simulink subsystem "AeroPropRefFranc"  (R2024b)
settings: Solver=VariableStepAuto  StartTime=0.0  StopTime=10.0  RelTol=1e-3
undefined symbols (not defined in the file or in its folder): ess, Force_b, Fprop_r, geom, H_b, Hdot_b, Moment_b, mot, mot2, mot3, mot4, Mprop_r, propel, propel2, propel3, propel4, pxf_diagram_options, SimIn, SimPar, tc, tc2, tc3, tc4
libraries: simulink x8, slpidlib x4, starslibAxisTransformations x2, libAxisTransformations x2
(part 4 of 10)

== system AeroPropRefFranc/Propulsion and Aerodynamic Forces and Moments/S-Function/Battery Model/powerplant/ess (battery)1/plant/parameter_out ==
  inport-ess_plant_soc_simu : Inport
  inport-ess_plant_curr_out_simu : Inport  Port=2
  inport-ess_plant_volt_out_simu : Inport  Port=3
  inport-ess_plant_voc_simu : Inport  Port=4
  inport-ess_plant_rint_simu : Inport  Port=5
  inport-ess_plant_rpol1_simu : Inport  Port=6
  inport-ess_plant_rpol2_simu : Inport  Port=7
  inport-ess_plant_curr_pol1_simu : Inport  Port=8
  inport-ess_plant_curr_pol2_simu : Inport  Port=9
  inport-ess_plant_heat_out_simu : Inport  Port=10
  inport-ess_plant_impedance_simu : Inport  Port=11
  Ground_1 : Ground
  Toworkspace-ess_plant_curr_out_simu : ToWorkspace  VariableName=ess_plant_curr_out_simu  SampleTime=pxf_diagram_options.workspace_sample_time
      settings: Decimation=pxf_diagram_options.decimation
  Toworkspace-ess_plant_curr_pol1_simu : ToWorkspace  VariableName=ess_plant_curr_pol1_simu  SampleTime=pxf_diagram_options.workspace_sample_time
      settings: Decimation=pxf_diagram_options.decimation
  Toworkspace-ess_plant_curr_pol2_simu : ToWorkspace  VariableName=ess_plant_curr_pol2_simu  SampleTime=pxf_diagram_options.workspace_sample_time
      settings: Decimation=pxf_diagram_options.decimation
  Toworkspace-ess_plant_heat_out_simu : ToWorkspace  VariableName=ess_plant_heat_out_simu  SampleTime=pxf_diagram_options.workspace_sample_time
      settings: Decimation=pxf_diagram_options.decimation
  Toworkspace-ess_plant_impedance_simu : ToWorkspace  VariableName=ess_plant_impedance_simu  SampleTime=pxf_diagram_options.workspace_sample_time
      settings: Decimation=pxf_diagram_options.decimation
  Toworkspace-ess_plant_rint_simu : ToWorkspace  VariableName=ess_plant_rint_simu  SampleTime=pxf_diagram_options.workspace_sample_time
      settings: Decimation=pxf_diagram_options.decimation
  Toworkspace-ess_plant_rpol1_simu : ToWorkspace  VariableName=ess_plant_rpol1_simu  SampleTime=pxf_diagram_options.workspace_sample_time
      settings: Decimation=pxf_diagram_options.decimation
  Toworkspace-ess_plant_rpol2_simu : ToWorkspace  VariableName=ess_plant_rpol2_simu  SampleTime=pxf_diagram_options.workspace_sample_time
      settings: Decimation=pxf_diagram_options.decimation
  Toworkspace-ess_plant_soc_simu : ToWorkspace  VariableName=ess_plant_soc_simu  SampleTime=pxf_diagram_options.workspace_sample_time
      settings: Decimation=pxf_diagram_options.decimation
  Toworkspace-ess_plant_voc_simu : ToWorkspace  VariableName=ess_plant_voc_simu  SampleTime=pxf_diagram_options.workspace_sample_time
      settings: Decimation=pxf_diagram_options.decimation
  Toworkspace-ess_plant_volt_out_simu : ToWorkspace  VariableName=ess_plant_volt_out_simu  SampleTime=pxf_diagram_options.workspace_sample_time
      settings: Decimation=pxf_diagram_options.decimation
  create_system_info_bus : BusCreator  Inputs=3
  outport-system_info_bus : Outport
  outport-plant_bus : Outport  Port=2
  wires:
  create_system_info_bus/1 -> outport-system_info_bus/1
  inport-ess_plant_soc_simu/1 -> create_system_info_bus/1, Toworkspace-ess_plant_soc_simu/1  "ess_plant_soc_simu"
  inport-ess_plant_heat_out_simu/1 -> Toworkspace-ess_plant_heat_out_simu/1
  inport-ess_plant_impedance_simu/1 -> Toworkspace-ess_plant_impedance_simu/1
  inport-ess_plant_curr_out_simu/1 -> create_system_info_bus/2, Toworkspace-ess_plant_curr_out_simu/1  "ess_plant_curr_out_simu"
  inport-ess_plant_volt_out_simu/1 -> create_system_info_bus/3, Toworkspace-ess_plant_volt_out_simu/1  "ess_plant_volt_out_simu"
  inport-ess_plant_voc_simu/1 -> Toworkspace-ess_plant_voc_simu/1
  inport-ess_plant_rint_simu/1 -> Toworkspace-ess_plant_rint_simu/1
  inport-ess_plant_rpol1_simu/1 -> Toworkspace-ess_plant_rpol1_simu/1
  inport-ess_plant_rpol2_simu/1 -> Toworkspace-ess_plant_rpol2_simu/1
  inport-ess_plant_curr_pol1_simu/1 -> Toworkspace-ess_plant_curr_pol1_simu/1
  inport-ess_plant_curr_pol2_simu/1 -> Toworkspace-ess_plant_curr_pol2_simu/1
  Ground_1/1 -> outport-plant_bus/1

== system AeroPropRefFranc/Propulsion and Aerodynamic Forces and Moments/S-Function/Battery Model/powerplant/ess (battery)1/plant/parameter_selection ==

== system AeroPropRefFranc/Propulsion and Aerodynamic Forces and Moments/S-Function/Battery Model/powerplant/mot/ctrl/cmd ==
  inport-main_info_bus-1 : Inport
  aInport--2 : Inport  Port=2
  aInport--3 : Inport  Port=3
  aInport--4 : Inport  Port=4
  Terminator_1 : Terminator
  Terminator_2 : Terminator
  Terminator_3 : Terminator
  mot_ctrl_cmd_map_Pelec_funTW_volt_in : Subsystem
  parameter_out : Subsystem
  parameter_selection : Subsystem
  outport-system_info_bus : Outport
  wires:
  aInport--4/1 -> Terminator_3/1
  aInport--3/1 -> Terminator_2/1
  aInport--2/1 -> Terminator_1/1
  parameter_selection/4(outport-mot_ctrl_cstr_trq_max_neg_simu-4) -> mot_ctrl_cmd_map_Pelec_funTW_volt_in/4(mot_ctrl_cstr_trq_max_neg_simu)
  parameter_selection/3(outport-mot_ctrl_cstr_trq_max_pos_simu-3) -> mot_ctrl_cmd_map_Pelec_funTW_volt_in/3(mot_ctrl_cstr_trq_max_pos_simu)
  parameter_selection/2(outport-mot_ctrl_trs_trq_simu-2) -> mot_ctrl_cmd_map_Pelec_funTW_volt_in/2(mot_ctrl_trs_trq_simu)
  parameter_selection/1(outport-mot_plant_spd_out_simu-1) -> mot_ctrl_cmd_map_Pelec_funTW_volt_in/1(mot_plant_spd_out_simu)
  mot_ctrl_cmd_map_Pelec_funTW_volt_in/1(mot_ctrl_cmd_simu) -> parameter_out/1(inport-mot_ctrl_cmd_simu)
  parameter_out/1(outport-system_info_bus) -> outport-system_info_bus/1
  inport-main_info_bus-1/1 -> parameter_selection/1(inport-main_info_bus-1)

== system AeroPropRefFranc/Propulsion and Aerodynamic Forces and Moments/S-Function/Battery Model/powerplant/mot/ctrl/cstr ==
  inport-main_info_bus-1 : Inport
  aInport--2 : Inport  Port=2
  aInport--3 : Inport  Port=3
  Terminator_1 : Terminator
  Terminator_2 : Terminator
  mot_ctrl_cstr_map_Pelec_funTW_volt_in : Subsystem
  parameter_out : Subsystem
  parameter_selection : Subsystem
  outport-system_info_bus : Outport
  outport-cstr_bus : Outport  Port=2
  wires:
  aInport--3/1 -> Terminator_2/1
  aInport--2/1 -> Terminator_1/1
  parameter_selection/2(outport-mot_plant_temp_coeff_simu-2) -> mot_ctrl_cstr_map_Pelec_funTW_volt_in/2(mot_plant_temp_coeff_simu)
  parameter_selection/1(outport-mot_plant_spd_out_simu-1) -> mot_ctrl_cstr_map_Pelec_funTW_volt_in/1(mot_plant_spd_out_simu)
  mot_ctrl_cstr_map_Pelec_funTW_volt_in/7(mot_ctrl_cstr_temp_coeff_simu) -> parameter_out/7(inport-mot_ctrl_cstr_temp_coeff_simu)
  mot_ctrl_cstr_map_Pelec_funTW_volt_in/6(mot_ctrl_cstr_trq_cont_neg_simu) -> parameter_out/6(inport-mot_ctrl_cstr_trq_cont_neg_simu)
  mot_ctrl_cstr_map_Pelec_funTW_volt_in/5(mot_ctrl_cstr_trq_cont_pos_simu) -> parameter_out/5(inport-mot_ctrl_cstr_trq_cont_pos_simu)
  mot_ctrl_cstr_map_Pelec_funTW_volt_in/4(mot_ctrl_cstr_trq_max_neg_simu) -> parameter_out/4(inport-mot_ctrl_cstr_trq_max_neg_simu)
  mot_ctrl_cstr_map_Pelec_funTW_volt_in/3(mot_ctrl_cstr_trq_pk_neg_simu) -> parameter_out/3(inport-mot_ctrl_cstr_trq_pk_neg_simu)
  mot_ctrl_cstr_map_Pelec_funTW_volt_in/2(mot_ctrl_cstr_trq_max_pos_simu) -> parameter_out/2(inport-mot_ctrl_cstr_trq_max_pos_simu)
  mot_ctrl_cstr_map_Pelec_funTW_volt_in/1(mot_ctrl_cstr_trq_pk_pos_simu) -> parameter_out/1(inport-mot_ctrl_cstr_trq_pk_pos_simu)
  parameter_out/2(outport-cstr_bus) -> outport-cstr_bus/1
  parameter_out/1(outport-system_info_bus) -> outport-system_info_bus/1
  inport-main_info_bus-1/1 -> parameter_selection/1(inport-main_info_bus-1)

== system AeroPropRefFranc/Propulsion and Aerodynamic Forces and Moments/S-Function/Battery Model/powerplant/mot/ctrl/dmd ==
  inport-main_info_bus-1 : Inport
  aInport--2 : Inport  Port=2
  Terminator_1 : Terminator
  mot_ctrl_dmd_uas : Subsystem
  parameter_out : Subsystem
  parameter_selection : Subsystem
  outport-system_info_bus : Outport
  outport-dmd_bus : Outport  Port=2
  wires:
  aInport--2/1 -> Terminator_1/1
  parameter_selection/5(outport-tc_plant_spd_in_simu-5) -> mot_ctrl_dmd_uas/5(tc_plant_spd_in_simu)
  parameter_selection/4(outport-propel_plant_speed_simu-4) -> mot_ctrl_dmd_uas/4(propel_plant_speed_simu)
  parameter_selection/3(outport-ess_ctrl_pwr_max_pro_simu-3) -> mot_ctrl_dmd_uas/3(ess_ctrl_pwr_max_pro_simu)
  parameter_selection/2(outport-env_plant_density_simu-2) -> mot_ctrl_dmd_uas/2(env_plant_density_simu)
  parameter_selection/1(outport-apc_ctrl_dt1_simu-1) -> mot_ctrl_dmd_uas/1(apc_ctrl_dt_simu)
  mot_ctrl_dmd_uas/2(mot_ctrl_ratedpwr_simu) -> parameter_out/2(inport-mot_ctrl_ratedpwr_simu)
  mot_ctrl_dmd_uas/1(mot_ctrl_trs_trq_simu) -> parameter_out/1(inport-mot_ctrl_trs_trq_simu)
  parameter_out/2(outport-dmd_bus) -> outport-dmd_bus/1
  parameter_out/1(outport-system_info_bus) -> outport-system_info_bus/1
  inport-main_info_bus-1/1 -> parameter_selection/1(inport-main_info_bus-1)

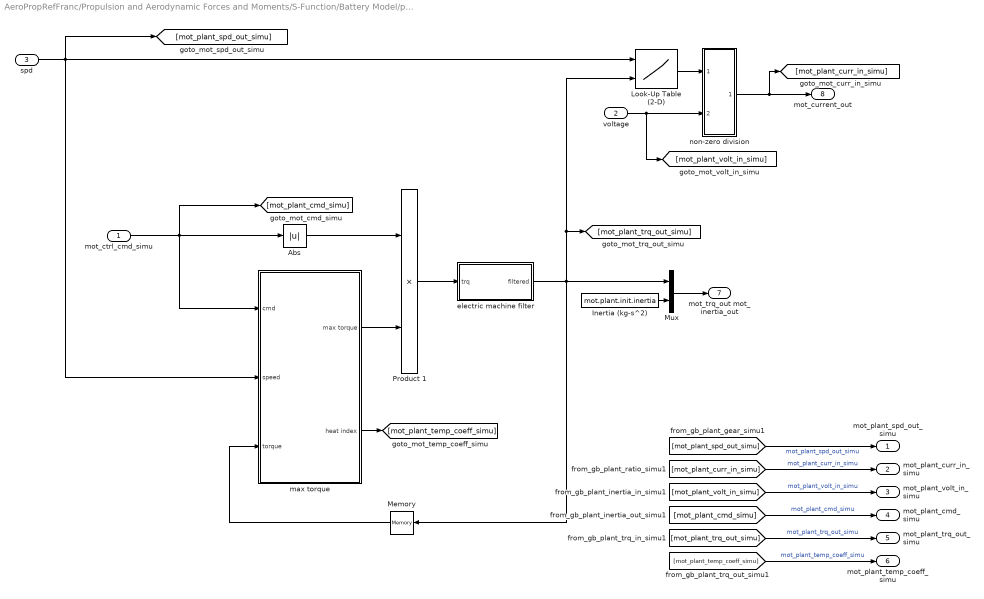
== system AeroPropRefFranc/Propulsion and Aerodynamic Forces and Moments/S-Function/Battery Model/powerplant/mot/plant/mot_plant_map_Pelec_funTW_volt_in ==
  mot_ctrl_cmd_simu : Inport
  voltage : Inport  Port=2
  spd : Inport  Port=3
  Abs : Abs
  Inertia (kg-s^2) : Constant  Value=mot.plant.init.inertia
  Look-Up Table (2-D) : Lookup2D  RowIndex=mot.plant.calc.pwr_elec.idx1_spd  ColumnIndex=mot.plant.calc.pwr_elec.idx2_trq  Table=mot.plant.calc.pwr_elec.map
  Memory : Memory
  Mux : Mux  Inputs=2
  Product 1 : Product  InputSameDT=on  SaturateOnIntegerOverflow=on  OutDataTypeStr=Inherit: Same as first input
  electric machine filter : Subsystem
  "max torque " : Subsystem
  non-zero division : Subsystem
      mask Display: disp('divider \n I1/I2')
  mot_plant_spd_out_simu : Outport
  mot_plant_curr_in_simu : Outport  Port=2
  mot_plant_volt_in_simu : Outport  Port=3
  mot_plant_cmd_simu : Outport  Port=4
  mot_plant_trq_out_simu : Outport  Port=5
  mot_plant_temp_coeff_simu : Outport  Port=6
  mot_trq_out mot_inertia_out : Outport  Port=7
  mot_current_out : Outport  Port=8
  wires:
  voltage/1 -> [mot_plant_volt_in_simu], non-zero division/2(In2)
  non-zero division/1(Out1) -> [mot_plant_curr_in_simu], mot_current_out/1
  "max torque "/2(heat index) -> [mot_plant_temp_coeff_simu]
  spd/1 -> Look-Up Table (2-D)/1, "max torque "/2(speed), [mot_plant_spd_out_simu]
  Mux/1 -> mot_trq_out mot_inertia_out/1
  Inertia (kg-s^2)/1 -> Mux/2
  mot_ctrl_cmd_simu/1 -> Abs/1, [mot_plant_cmd_simu], "max torque "/1(cmd)
  Memory/1 -> "max torque "/3(torque)
  Abs/1 -> Product 1/1
  Product 1/1 -> electric machine filter/1(trq)
  "max torque "/1(max torque) -> Product 1/2
  electric machine filter/1(filtered) -> Look-Up Table (2-D)/2, [mot_plant_trq_out_simu], Memory/1, Mux/1
  [mot_plant_spd_out_simu] -> mot_plant_spd_out_simu/1  "mot_plant_spd_out_simu"
  [mot_plant_curr_in_simu] -> mot_plant_curr_in_simu/1  "mot_plant_curr_in_simu"
  [mot_plant_volt_in_simu] -> mot_plant_volt_in_simu/1  "mot_plant_volt_in_simu"
  [mot_plant_cmd_simu] -> mot_plant_cmd_simu/1  "mot_plant_cmd_simu"
  [mot_plant_trq_out_simu] -> mot_plant_trq_out_simu/1  "mot_plant_trq_out_simu"
  [mot_plant_temp_coeff_simu] -> mot_plant_temp_coeff_simu/1  "mot_plant_temp_coeff_simu"
  Look-Up Table (2-D)/1 -> non-zero division/1(In1)

== system AeroPropRefFranc/Propulsion and Aerodynamic Forces and Moments/S-Function/Battery Model/powerplant/mot/plant/parameter_out ==
  inport-mot_plant_spd_out_simu : Inport
  inport-mot_plant_curr_in_simu : Inport  Port=2
  inport-mot_plant_volt_in_simu : Inport  Port=3
  inport-mot_plant_cmd_simu : Inport  Port=4
  inport-mot_plant_trq_out_simu : Inport  Port=5
  inport-mot_plant_temp_coeff_simu : Inport  Port=6
  Ground_1 : Ground
  Toworkspace-mot_plant_cmd_simu : ToWorkspace  VariableName=mot_plant_cmd_simu  SampleTime=pxf_diagram_options.workspace_sample_time
      settings: Decimation=pxf_diagram_options.decimation
  Toworkspace-mot_plant_curr_in_simu : ToWorkspace  VariableName=mot_plant_curr_in_simu  SampleTime=pxf_diagram_options.workspace_sample_time
      settings: Decimation=pxf_diagram_options.decimation
  Toworkspace-mot_plant_spd_out_simu : ToWorkspace  VariableName=mot_plant_spd_out_simu  SampleTime=pxf_diagram_options.workspace_sample_time
      settings: Decimation=pxf_diagram_options.decimation
  Toworkspace-mot_plant_temp_coeff_simu : ToWorkspace  VariableName=mot_plant_temp_coeff_simu  SampleTime=pxf_diagram_options.workspace_sample_time
      settings: Decimation=pxf_diagram_options.decimation
  Toworkspace-mot_plant_trq_out_simu : ToWorkspace  VariableName=mot_plant_trq_out_simu  SampleTime=pxf_diagram_options.workspace_sample_time
      settings: Decimation=pxf_diagram_options.decimation
  Toworkspace-mot_plant_volt_in_simu : ToWorkspace  VariableName=mot_plant_volt_in_simu  SampleTime=pxf_diagram_options.workspace_sample_time
      settings: Decimation=pxf_diagram_options.decimation
  create_system_info_bus : BusCreator  Inputs=2
  outport-system_info_bus : Outport
  outport-plant_bus : Outport  Port=2
  wires:
  Ground_1/1 -> outport-plant_bus/1
  inport-mot_plant_temp_coeff_simu/1 -> Toworkspace-mot_plant_temp_coeff_simu/1, create_system_info_bus/2  "mot_plant_temp_coeff_simu"
  inport-mot_plant_trq_out_simu/1 -> Toworkspace-mot_plant_trq_out_simu/1
  inport-mot_plant_cmd_simu/1 -> Toworkspace-mot_plant_cmd_simu/1
  inport-mot_plant_volt_in_simu/1 -> Toworkspace-mot_plant_volt_in_simu/1
  inport-mot_plant_curr_in_simu/1 -> Toworkspace-mot_plant_curr_in_simu/1
  inport-mot_plant_spd_out_simu/1 -> Toworkspace-mot_plant_spd_out_simu/1, create_system_info_bus/1  "mot_plant_spd_out_simu"
  create_system_info_bus/1 -> outport-system_info_bus/1

== system AeroPropRefFranc/Propulsion and Aerodynamic Forces and Moments/S-Function/Battery Model/powerplant/mot/plant/parameter_selection ==
  Inport_1 : Inport
  inport-ctrl_bus-2 : Inport  Port=2
  Terminator_1 : Terminator
  select_ctrl_bus : BusSelector  OutputSignals=mot_ctrl_cmd_simu
  outport-mot_ctrl_cmd_simu-1 : Outport
  wires:
  Inport_1/1 -> Terminator_1/1
  select_ctrl_bus/1 -> outport-mot_ctrl_cmd_simu-1/1  "<mot_ctrl_cmd_simu>"
  inport-ctrl_bus-2/1 -> select_ctrl_bus/1

== system AeroPropRefFranc/Propulsion and Aerodynamic Forces and Moments/S-Function/Battery Model/powerplant/mot2/ctrl/cmd ==
  inport-main_info_bus-1 : Inport
  aInport--2 : Inport  Port=2
  aInport--3 : Inport  Port=3
  aInport--4 : Inport  Port=4
  Terminator_1 : Terminator
  Terminator_2 : Terminator
  Terminator_3 : Terminator
  mot2_ctrl_cmd_map_Pelec_funTW_volt_in : Subsystem
  parameter_out : Subsystem
  parameter_selection : Subsystem
  outport-system_info_bus : Outport
  wires:
  aInport--4/1 -> Terminator_3/1
  aInport--3/1 -> Terminator_2/1
  aInport--2/1 -> Terminator_1/1
  parameter_selection/4(outport-mot2_ctrl_cstr_trq_max_neg_simu-4) -> mot2_ctrl_cmd_map_Pelec_funTW_volt_in/4(mot_ctrl_cstr_trq_max_neg_simu)
  parameter_selection/3(outport-mot2_ctrl_cstr_trq_max_pos_simu-3) -> mot2_ctrl_cmd_map_Pelec_funTW_volt_in/3(mot_ctrl_cstr_trq_max_pos_simu)
  parameter_selection/2(outport-mot2_ctrl_trs_trq_simu-2) -> mot2_ctrl_cmd_map_Pelec_funTW_volt_in/2(mot_ctrl_trs_trq_simu)
  parameter_selection/1(outport-mot2_plant_spd_out_simu-1) -> mot2_ctrl_cmd_map_Pelec_funTW_volt_in/1(mot_plant_spd_out_simu)
  mot2_ctrl_cmd_map_Pelec_funTW_volt_in/1(mot_ctrl_cmd_simu) -> parameter_out/1(inport-mot2_ctrl_cmd_simu)
  parameter_out/1(outport-system_info_bus) -> outport-system_info_bus/1
  inport-main_info_bus-1/1 -> parameter_selection/1(inport-main_info_bus-1)

== system AeroPropRefFranc/Propulsion and Aerodynamic Forces and Moments/S-Function/Battery Model/powerplant/mot2/ctrl/cstr ==
  inport-main_info_bus-1 : Inport
  aInport--2 : Inport  Port=2
  aInport--3 : Inport  Port=3
  Terminator_1 : Terminator
  Terminator_2 : Terminator
  mot2_ctrl_cstr_map_Pelec_funTW_volt_in : Subsystem
  parameter_out : Subsystem
  parameter_selection : Subsystem
  outport-system_info_bus : Outport
  outport-cstr_bus : Outport  Port=2
  wires:
  aInport--3/1 -> Terminator_2/1
  aInport--2/1 -> Terminator_1/1
  parameter_selection/2(outport-mot2_plant_temp_coeff_simu-2) -> mot2_ctrl_cstr_map_Pelec_funTW_volt_in/2(mot_plant_temp_coeff_simu)
  parameter_selection/1(outport-mot2_plant_spd_out_simu-1) -> mot2_ctrl_cstr_map_Pelec_funTW_volt_in/1(mot_plant_spd_out_simu)
  mot2_ctrl_cstr_map_Pelec_funTW_volt_in/7(mot_ctrl_cstr_temp_coeff_simu) -> parameter_out/7(inport-mot2_ctrl_cstr_temp_coeff_simu)
  mot2_ctrl_cstr_map_Pelec_funTW_volt_in/6(mot_ctrl_cstr_trq_cont_neg_simu) -> parameter_out/6(inport-mot2_ctrl_cstr_trq_cont_neg_simu)
  mot2_ctrl_cstr_map_Pelec_funTW_volt_in/5(mot_ctrl_cstr_trq_cont_pos_simu) -> parameter_out/5(inport-mot2_ctrl_cstr_trq_cont_pos_simu)
  mot2_ctrl_cstr_map_Pelec_funTW_volt_in/4(mot_ctrl_cstr_trq_max_neg_simu) -> parameter_out/4(inport-mot2_ctrl_cstr_trq_max_neg_simu)
  mot2_ctrl_cstr_map_Pelec_funTW_volt_in/3(mot_ctrl_cstr_trq_pk_neg_simu) -> parameter_out/3(inport-mot2_ctrl_cstr_trq_pk_neg_simu)
  mot2_ctrl_cstr_map_Pelec_funTW_volt_in/2(mot_ctrl_cstr_trq_max_pos_simu) -> parameter_out/2(inport-mot2_ctrl_cstr_trq_max_pos_simu)
  mot2_ctrl_cstr_map_Pelec_funTW_volt_in/1(mot_ctrl_cstr_trq_pk_pos_simu) -> parameter_out/1(inport-mot2_ctrl_cstr_trq_pk_pos_simu)
  parameter_out/2(outport-cstr_bus) -> outport-cstr_bus/1
  parameter_out/1(outport-system_info_bus) -> outport-system_info_bus/1
  inport-main_info_bus-1/1 -> parameter_selection/1(inport-main_info_bus-1)

== system AeroPropRefFranc/Propulsion and Aerodynamic Forces and Moments/S-Function/Battery Model/powerplant/mot2/ctrl/dmd ==
  inport-main_info_bus-1 : Inport
  aInport--2 : Inport  Port=2
  Terminator_1 : Terminator
  mot2_ctrl_dmd_uas : Subsystem
  parameter_out : Subsystem
  parameter_selection : Subsystem
  outport-system_info_bus : Outport
  outport-dmd_bus : Outport  Port=2
  wires:
  aInport--2/1 -> Terminator_1/1
  parameter_selection/5(outport-tc2_plant_spd_in_simu-5) -> mot2_ctrl_dmd_uas/5(tc_plant_spd_in_simu)
  parameter_selection/4(outport-propel2_plant_speed_simu-4) -> mot2_ctrl_dmd_uas/4(propel_plant_speed_simu)
  parameter_selection/3(outport-ess_ctrl_pwr_max_pro_simu-3) -> mot2_ctrl_dmd_uas/3(ess_ctrl_pwr_max_pro_simu)
  parameter_selection/2(outport-env_plant_density_simu-2) -> mot2_ctrl_dmd_uas/2(env_plant_density_simu)
  parameter_selection/1(outport-apc_ctrl_dt2_simu-1) -> mot2_ctrl_dmd_uas/1(apc_ctrl_dt_simu)
  mot2_ctrl_dmd_uas/2(mot_ctrl_ratedpwr_simu) -> parameter_out/2(inport-mot2_ctrl_ratedpwr_simu)
  mot2_ctrl_dmd_uas/1(mot_ctrl_trs_trq_simu) -> parameter_out/1(inport-mot2_ctrl_trs_trq_simu)
  parameter_out/2(outport-dmd_bus) -> outport-dmd_bus/1
  parameter_out/1(outport-system_info_bus) -> outport-system_info_bus/1
  inport-main_info_bus-1/1 -> parameter_selection/1(inport-main_info_bus-1)

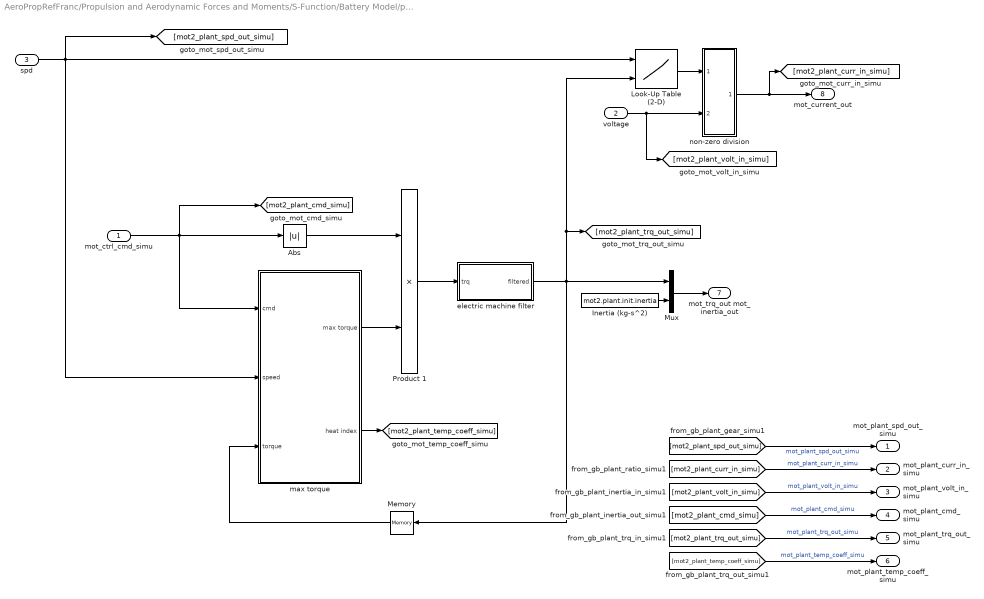
== system AeroPropRefFranc/Propulsion and Aerodynamic Forces and Moments/S-Function/Battery Model/powerplant/mot2/plant/mot2_plant_map_Pelec_funTW_volt_in ==
  mot_ctrl_cmd_simu : Inport
  voltage : Inport  Port=2
  spd : Inport  Port=3
  Abs : Abs
  Inertia (kg-s^2) : Constant  Value=mot2.plant.init.inertia
  Look-Up Table (2-D) : Lookup2D  RowIndex=mot2.plant.calc.pwr_elec.idx1_spd  ColumnIndex=mot2.plant.calc.pwr_elec.idx2_trq  Table=mot2.plant.calc.pwr_elec.map
  Memory : Memory
  Mux : Mux  Inputs=2
  Product 1 : Product  InputSameDT=on  SaturateOnIntegerOverflow=on  OutDataTypeStr=Inherit: Same as first input
  electric machine filter : Subsystem
  "max torque " : Subsystem
  non-zero division : Subsystem
      mask Display: disp('divider \n I1/I2')
  mot_plant_spd_out_simu : Outport
  mot_plant_curr_in_simu : Outport  Port=2
  mot_plant_volt_in_simu : Outport  Port=3
  mot_plant_cmd_simu : Outport  Port=4
  mot_plant_trq_out_simu : Outport  Port=5
  mot_plant_temp_coeff_simu : Outport  Port=6
  mot_trq_out mot_inertia_out : Outport  Port=7
  mot_current_out : Outport  Port=8
  wires:
  voltage/1 -> [mot2_plant_volt_in_simu], non-zero division/2(In2)
  non-zero division/1(Out1) -> [mot2_plant_curr_in_simu], mot_current_out/1
  "max torque "/2(heat index) -> [mot2_plant_temp_coeff_simu]
  spd/1 -> Look-Up Table (2-D)/1, "max torque "/2(speed), [mot2_plant_spd_out_simu]
  Mux/1 -> mot_trq_out mot_inertia_out/1
  Inertia (kg-s^2)/1 -> Mux/2
  mot_ctrl_cmd_simu/1 -> Abs/1, [mot2_plant_cmd_simu], "max torque "/1(cmd)
  Memory/1 -> "max torque "/3(torque)
  Abs/1 -> Product 1/1
  Product 1/1 -> electric machine filter/1(trq)
  "max torque "/1(max torque) -> Product 1/2
  electric machine filter/1(filtered) -> Look-Up Table (2-D)/2, [mot2_plant_trq_out_simu], Memory/1, Mux/1
  [mot2_plant_spd_out_simu] -> mot_plant_spd_out_simu/1  "mot_plant_spd_out_simu"
  [mot2_plant_curr_in_simu] -> mot_plant_curr_in_simu/1  "mot_plant_curr_in_simu"
  [mot2_plant_volt_in_simu] -> mot_plant_volt_in_simu/1  "mot_plant_volt_in_simu"
  [mot2_plant_cmd_simu] -> mot_plant_cmd_simu/1  "mot_plant_cmd_simu"
  [mot2_plant_trq_out_simu] -> mot_plant_trq_out_simu/1  "mot_plant_trq_out_simu"
  [mot2_plant_temp_coeff_simu] -> mot_plant_temp_coeff_simu/1  "mot_plant_temp_coeff_simu"
  Look-Up Table (2-D)/1 -> non-zero division/1(In1)

== system AeroPropRefFranc/Propulsion and Aerodynamic Forces and Moments/S-Function/Battery Model/powerplant/mot2/plant/parameter_out ==
  inport-mot2_plant_spd_out_simu : Inport
  inport-mot2_plant_curr_in_simu : Inport  Port=2
  inport-mot2_plant_volt_in_simu : Inport  Port=3
  inport-mot2_plant_cmd_simu : Inport  Port=4
  inport-mot2_plant_trq_out_simu : Inport  Port=5
  inport-mot2_plant_temp_coeff_simu : Inport  Port=6
  Ground_1 : Ground
  Toworkspace-mot2_plant_cmd_simu : ToWorkspace  VariableName=mot2_plant_cmd_simu  SampleTime=pxf_diagram_options.workspace_sample_time
      settings: Decimation=pxf_diagram_options.decimation
  Toworkspace-mot2_plant_curr_in_simu : ToWorkspace  VariableName=mot2_plant_curr_in_simu  SampleTime=pxf_diagram_options.workspace_sample_time
      settings: Decimation=pxf_diagram_options.decimation
  Toworkspace-mot2_plant_spd_out_simu : ToWorkspace  VariableName=mot2_plant_spd_out_simu  SampleTime=pxf_diagram_options.workspace_sample_time
      settings: Decimation=pxf_diagram_options.decimation
  Toworkspace-mot2_plant_temp_coeff_simu : ToWorkspace  VariableName=mot2_plant_temp_coeff_simu  SampleTime=pxf_diagram_options.workspace_sample_time
      settings: Decimation=pxf_diagram_options.decimation
  Toworkspace-mot2_plant_trq_out_simu : ToWorkspace  VariableName=mot2_plant_trq_out_simu  SampleTime=pxf_diagram_options.workspace_sample_time
      settings: Decimation=pxf_diagram_options.decimation
  Toworkspace-mot2_plant_volt_in_simu : ToWorkspace  VariableName=mot2_plant_volt_in_simu  SampleTime=pxf_diagram_options.workspace_sample_time
      settings: Decimation=pxf_diagram_options.decimation
  create_system_info_bus : BusCreator  Inputs=2
  outport-system_info_bus : Outport
  outport-plant_bus : Outport  Port=2
  wires:
  Ground_1/1 -> outport-plant_bus/1
  inport-mot2_plant_temp_coeff_simu/1 -> Toworkspace-mot2_plant_temp_coeff_simu/1, create_system_info_bus/2  "mot2_plant_temp_coeff_simu"
  inport-mot2_plant_trq_out_simu/1 -> Toworkspace-mot2_plant_trq_out_simu/1
  inport-mot2_plant_cmd_simu/1 -> Toworkspace-mot2_plant_cmd_simu/1
  inport-mot2_plant_volt_in_simu/1 -> Toworkspace-mot2_plant_volt_in_simu/1
  inport-mot2_plant_curr_in_simu/1 -> Toworkspace-mot2_plant_curr_in_simu/1
  inport-mot2_plant_spd_out_simu/1 -> Toworkspace-mot2_plant_spd_out_simu/1, create_system_info_bus/1  "mot2_plant_spd_out_simu"
  create_system_info_bus/1 -> outport-system_info_bus/1

== system AeroPropRefFranc/Propulsion and Aerodynamic Forces and Moments/S-Function/Battery Model/powerplant/mot2/plant/parameter_selection ==
  Inport_1 : Inport
  inport-ctrl_bus-2 : Inport  Port=2
  Terminator_1 : Terminator
  select_ctrl_bus : BusSelector  OutputSignals=mot2_ctrl_cmd_simu
  outport-mot2_ctrl_cmd_simu-1 : Outport
  wires:
  Inport_1/1 -> Terminator_1/1
  select_ctrl_bus/1 -> outport-mot2_ctrl_cmd_simu-1/1  "<mot2_ctrl_cmd_simu>"
  inport-ctrl_bus-2/1 -> select_ctrl_bus/1

== system AeroPropRefFranc/Propulsion and Aerodynamic Forces and Moments/S-Function/Battery Model/powerplant/mot3/ctrl/cmd ==
  inport-main_info_bus-1 : Inport
  aInport--2 : Inport  Port=2
  aInport--3 : Inport  Port=3
  aInport--4 : Inport  Port=4
  Terminator_1 : Terminator
  Terminator_2 : Terminator
  Terminator_3 : Terminator
  mot3_ctrl_cmd_map_Pelec_funTW_volt_in : Subsystem
  parameter_out : Subsystem
  parameter_selection : Subsystem
  outport-system_info_bus : Outport
  wires:
  aInport--4/1 -> Terminator_3/1
  aInport--3/1 -> Terminator_2/1
  aInport--2/1 -> Terminator_1/1
  parameter_selection/4(outport-mot3_ctrl_cstr_trq_max_neg_simu-4) -> mot3_ctrl_cmd_map_Pelec_funTW_volt_in/4(mot_ctrl_cstr_trq_max_neg_simu)
  parameter_selection/3(outport-mot3_ctrl_cstr_trq_max_pos_simu-3) -> mot3_ctrl_cmd_map_Pelec_funTW_volt_in/3(mot_ctrl_cstr_trq_max_pos_simu)
  parameter_selection/2(outport-mot3_ctrl_trs_trq_simu-2) -> mot3_ctrl_cmd_map_Pelec_funTW_volt_in/2(mot_ctrl_trs_trq_simu)
  parameter_selection/1(outport-mot3_plant_spd_out_simu-1) -> mot3_ctrl_cmd_map_Pelec_funTW_volt_in/1(mot_plant_spd_out_simu)
  mot3_ctrl_cmd_map_Pelec_funTW_volt_in/1(mot_ctrl_cmd_simu) -> parameter_out/1(inport-mot3_ctrl_cmd_simu)
  parameter_out/1(outport-system_info_bus) -> outport-system_info_bus/1
  inport-main_info_bus-1/1 -> parameter_selection/1(inport-main_info_bus-1)

== system AeroPropRefFranc/Propulsion and Aerodynamic Forces and Moments/S-Function/Battery Model/powerplant/mot3/ctrl/cstr ==
  inport-main_info_bus-1 : Inport
  aInport--2 : Inport  Port=2
  aInport--3 : Inport  Port=3
  Terminator_1 : Terminator
  Terminator_2 : Terminator
  mot3_ctrl_cstr_map_Pelec_funTW_volt_in : Subsystem
  parameter_out : Subsystem
  parameter_selection : Subsystem
  outport-system_info_bus : Outport
  outport-cstr_bus : Outport  Port=2
  wires:
  aInport--3/1 -> Terminator_2/1
  aInport--2/1 -> Terminator_1/1
  parameter_selection/2(outport-mot3_plant_temp_coeff_simu-2) -> mot3_ctrl_cstr_map_Pelec_funTW_volt_in/2(mot_plant_temp_coeff_simu)
  parameter_selection/1(outport-mot3_plant_spd_out_simu-1) -> mot3_ctrl_cstr_map_Pelec_funTW_volt_in/1(mot_plant_spd_out_simu)
  mot3_ctrl_cstr_map_Pelec_funTW_volt_in/7(mot_ctrl_cstr_temp_coeff_simu) -> parameter_out/7(inport-mot3_ctrl_cstr_temp_coeff_simu)
  mot3_ctrl_cstr_map_Pelec_funTW_volt_in/6(mot_ctrl_cstr_trq_cont_neg_simu) -> parameter_out/6(inport-mot3_ctrl_cstr_trq_cont_neg_simu)
  mot3_ctrl_cstr_map_Pelec_funTW_volt_in/5(mot_ctrl_cstr_trq_cont_pos_simu) -> parameter_out/5(inport-mot3_ctrl_cstr_trq_cont_pos_simu)
  mot3_ctrl_cstr_map_Pelec_funTW_volt_in/4(mot_ctrl_cstr_trq_max_neg_simu) -> parameter_out/4(inport-mot3_ctrl_cstr_trq_max_neg_simu)
  mot3_ctrl_cstr_map_Pelec_funTW_volt_in/3(mot_ctrl_cstr_trq_pk_neg_simu) -> parameter_out/3(inport-mot3_ctrl_cstr_trq_pk_neg_simu)
  mot3_ctrl_cstr_map_Pelec_funTW_volt_in/2(mot_ctrl_cstr_trq_max_pos_simu) -> parameter_out/2(inport-mot3_ctrl_cstr_trq_max_pos_simu)
  mot3_ctrl_cstr_map_Pelec_funTW_volt_in/1(mot_ctrl_cstr_trq_pk_pos_simu) -> parameter_out/1(inport-mot3_ctrl_cstr_trq_pk_pos_simu)
  parameter_out/2(outport-cstr_bus) -> outport-cstr_bus/1
  parameter_out/1(outport-system_info_bus) -> outport-system_info_bus/1
  inport-main_info_bus-1/1 -> parameter_selection/1(inport-main_info_bus-1)

== system AeroPropRefFranc/Propulsion and Aerodynamic Forces and Moments/S-Function/Battery Model/powerplant/mot3/ctrl/dmd ==
  inport-main_info_bus-1 : Inport
  aInport--2 : Inport  Port=2
  Terminator_1 : Terminator
  mot3_ctrl_dmd_uas : Subsystem
  parameter_out : Subsystem
  parameter_selection : Subsystem
  outport-system_info_bus : Outport
  outport-dmd_bus : Outport  Port=2
  wires:
  aInport--2/1 -> Terminator_1/1
  parameter_selection/5(outport-tc3_plant_spd_in_simu-5) -> mot3_ctrl_dmd_uas/5(tc_plant_spd_in_simu)
  parameter_selection/4(outport-propel3_plant_speed_simu-4) -> mot3_ctrl_dmd_uas/4(propel_plant_speed_simu)
  parameter_selection/3(outport-ess_ctrl_pwr_max_pro_simu-3) -> mot3_ctrl_dmd_uas/3(ess_ctrl_pwr_max_pro_simu)
  parameter_selection/2(outport-env_plant_density_simu-2) -> mot3_ctrl_dmd_uas/2(env_plant_density_simu)
  parameter_selection/1(outport-apc_ctrl_dt3_simu-1) -> mot3_ctrl_dmd_uas/1(apc_ctrl_dt_simu)
  mot3_ctrl_dmd_uas/2(mot_ctrl_ratedpwr_simu) -> parameter_out/2(inport-mot3_ctrl_ratedpwr_simu)
  mot3_ctrl_dmd_uas/1(mot_ctrl_trs_trq_simu) -> parameter_out/1(inport-mot3_ctrl_trs_trq_simu)
  parameter_out/2(outport-dmd_bus) -> outport-dmd_bus/1
  parameter_out/1(outport-system_info_bus) -> outport-system_info_bus/1
  inport-main_info_bus-1/1 -> parameter_selection/1(inport-main_info_bus-1)

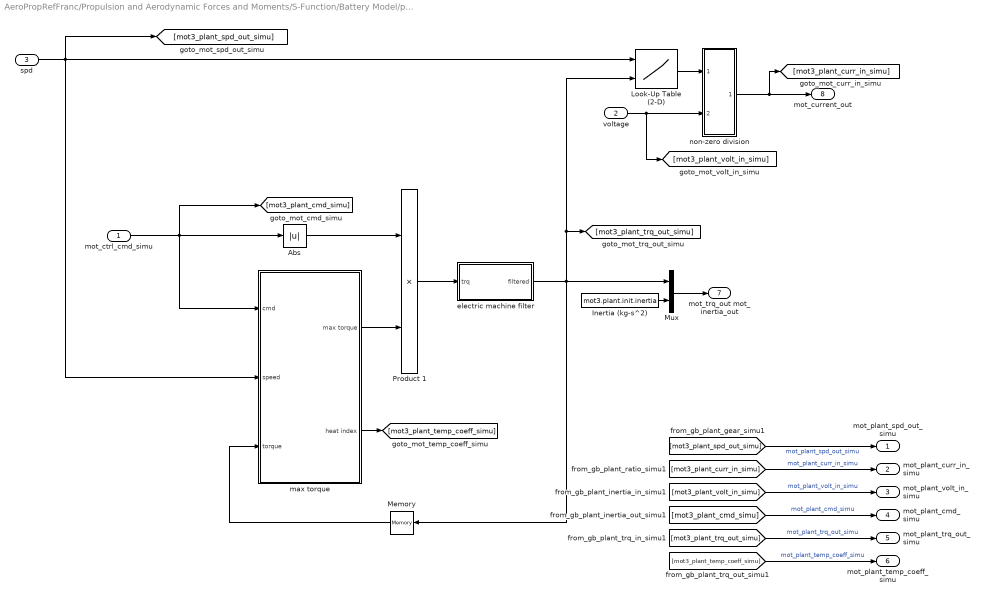
== system AeroPropRefFranc/Propulsion and Aerodynamic Forces and Moments/S-Function/Battery Model/powerplant/mot3/plant/mot3_plant_map_Pelec_funTW_volt_in ==
  mot_ctrl_cmd_simu : Inport
  voltage : Inport  Port=2
  spd : Inport  Port=3
  Abs : Abs
  Inertia (kg-s^2) : Constant  Value=mot3.plant.init.inertia
  Look-Up Table (2-D) : Lookup2D  RowIndex=mot3.plant.calc.pwr_elec.idx1_spd  ColumnIndex=mot3.plant.calc.pwr_elec.idx2_trq  Table=mot3.plant.calc.pwr_elec.map
  Memory : Memory
  Mux : Mux  Inputs=2
  Product 1 : Product  InputSameDT=on  SaturateOnIntegerOverflow=on  OutDataTypeStr=Inherit: Same as first input
  electric machine filter : Subsystem
  "max torque " : Subsystem
  non-zero division : Subsystem
      mask Display: disp('divider \n I1/I2')
  mot_plant_spd_out_simu : Outport
  mot_plant_curr_in_simu : Outport  Port=2
  mot_plant_volt_in_simu : Outport  Port=3
  mot_plant_cmd_simu : Outport  Port=4
  mot_plant_trq_out_simu : Outport  Port=5
  mot_plant_temp_coeff_simu : Outport  Port=6
  mot_trq_out mot_inertia_out : Outport  Port=7
  mot_current_out : Outport  Port=8
  wires:
  voltage/1 -> [mot3_plant_volt_in_simu], non-zero division/2(In2)
  non-zero division/1(Out1) -> [mot3_plant_curr_in_simu], mot_current_out/1
  "max torque "/2(heat index) -> [mot3_plant_temp_coeff_simu]
  spd/1 -> Look-Up Table (2-D)/1, "max torque "/2(speed), [mot3_plant_spd_out_simu]
  Mux/1 -> mot_trq_out mot_inertia_out/1
  Inertia (kg-s^2)/1 -> Mux/2
  mot_ctrl_cmd_simu/1 -> Abs/1, [mot3_plant_cmd_simu], "max torque "/1(cmd)
  Memory/1 -> "max torque "/3(torque)
  Abs/1 -> Product 1/1
  Product 1/1 -> electric machine filter/1(trq)
  "max torque "/1(max torque) -> Product 1/2
  electric machine filter/1(filtered) -> Look-Up Table (2-D)/2, [mot3_plant_trq_out_simu], Memory/1, Mux/1
  [mot3_plant_spd_out_simu] -> mot_plant_spd_out_simu/1  "mot_plant_spd_out_simu"
  [mot3_plant_curr_in_simu] -> mot_plant_curr_in_simu/1  "mot_plant_curr_in_simu"
  [mot3_plant_volt_in_simu] -> mot_plant_volt_in_simu/1  "mot_plant_volt_in_simu"
  [mot3_plant_cmd_simu] -> mot_plant_cmd_simu/1  "mot_plant_cmd_simu"
  [mot3_plant_trq_out_simu] -> mot_plant_trq_out_simu/1  "mot_plant_trq_out_simu"
  [mot3_plant_temp_coeff_simu] -> mot_plant_temp_coeff_simu/1  "mot_plant_temp_coeff_simu"
  Look-Up Table (2-D)/1 -> non-zero division/1(In1)

== system AeroPropRefFranc/Propulsion and Aerodynamic Forces and Moments/S-Function/Battery Model/powerplant/mot3/plant/parameter_out ==
  inport-mot3_plant_spd_out_simu : Inport
  inport-mot3_plant_curr_in_simu : Inport  Port=2
  inport-mot3_plant_volt_in_simu : Inport  Port=3
  inport-mot3_plant_cmd_simu : Inport  Port=4
  inport-mot3_plant_trq_out_simu : Inport  Port=5
  inport-mot3_plant_temp_coeff_simu : Inport  Port=6
  Ground_1 : Ground
  Toworkspace-mot3_plant_cmd_simu : ToWorkspace  VariableName=mot3_plant_cmd_simu  SampleTime=pxf_diagram_options.workspace_sample_time
      settings: Decimation=pxf_diagram_options.decimation
  Toworkspace-mot3_plant_curr_in_simu : ToWorkspace  VariableName=mot3_plant_curr_in_simu  SampleTime=pxf_diagram_options.workspace_sample_time
      settings: Decimation=pxf_diagram_options.decimation
  Toworkspace-mot3_plant_spd_out_simu : ToWorkspace  VariableName=mot3_plant_spd_out_simu  SampleTime=pxf_diagram_options.workspace_sample_time
      settings: Decimation=pxf_diagram_options.decimation
  Toworkspace-mot3_plant_temp_coeff_simu : ToWorkspace  VariableName=mot3_plant_temp_coeff_simu  SampleTime=pxf_diagram_options.workspace_sample_time
      settings: Decimation=pxf_diagram_options.decimation
  Toworkspace-mot3_plant_trq_out_simu : ToWorkspace  VariableName=mot3_plant_trq_out_simu  SampleTime=pxf_diagram_options.workspace_sample_time
      settings: Decimation=pxf_diagram_options.decimation
  Toworkspace-mot3_plant_volt_in_simu : ToWorkspace  VariableName=mot3_plant_volt_in_simu  SampleTime=pxf_diagram_options.workspace_sample_time
      settings: Decimation=pxf_diagram_options.decimation
  create_system_info_bus : BusCreator  Inputs=2
  outport-system_info_bus : Outport
  outport-plant_bus : Outport  Port=2
  wires:
  Ground_1/1 -> outport-plant_bus/1
  inport-mot3_plant_temp_coeff_simu/1 -> Toworkspace-mot3_plant_temp_coeff_simu/1, create_system_info_bus/2  "mot3_plant_temp_coeff_simu"
  inport-mot3_plant_trq_out_simu/1 -> Toworkspace-mot3_plant_trq_out_simu/1
  inport-mot3_plant_cmd_simu/1 -> Toworkspace-mot3_plant_cmd_simu/1
  inport-mot3_plant_volt_in_simu/1 -> Toworkspace-mot3_plant_volt_in_simu/1
  inport-mot3_plant_curr_in_simu/1 -> Toworkspace-mot3_plant_curr_in_simu/1
  inport-mot3_plant_spd_out_simu/1 -> Toworkspace-mot3_plant_spd_out_simu/1, create_system_info_bus/1  "mot3_plant_spd_out_simu"
  create_system_info_bus/1 -> outport-system_info_bus/1

== system AeroPropRefFranc/Propulsion and Aerodynamic Forces and Moments/S-Function/Battery Model/powerplant/mot3/plant/parameter_selection ==
  Inport_1 : Inport
  inport-ctrl_bus-2 : Inport  Port=2
  Terminator_1 : Terminator
  select_ctrl_bus : BusSelector  OutputSignals=mot3_ctrl_cmd_simu
  outport-mot3_ctrl_cmd_simu-1 : Outport
  wires:
  Inport_1/1 -> Terminator_1/1
  select_ctrl_bus/1 -> outport-mot3_ctrl_cmd_simu-1/1  "<mot3_ctrl_cmd_simu>"
  inport-ctrl_bus-2/1 -> select_ctrl_bus/1

== system AeroPropRefFranc/Propulsion and Aerodynamic Forces and Moments/S-Function/Battery Model/powerplant/mot4/ctrl/cmd ==
  inport-main_info_bus-1 : Inport
  aInport--2 : Inport  Port=2
  aInport--3 : Inport  Port=3
  aInport--4 : Inport  Port=4
  Terminator_1 : Terminator
  Terminator_2 : Terminator
  Terminator_3 : Terminator
  mot4_ctrl_cmd_map_Pelec_funTW_volt_in : Subsystem
  parameter_out : Subsystem
  parameter_selection : Subsystem
  outport-system_info_bus : Outport
  wires:
  aInport--4/1 -> Terminator_3/1
  aInport--3/1 -> Terminator_2/1
  aInport--2/1 -> Terminator_1/1
  parameter_selection/4(outport-mot4_ctrl_cstr_trq_max_neg_simu-4) -> mot4_ctrl_cmd_map_Pelec_funTW_volt_in/4(mot_ctrl_cstr_trq_max_neg_simu)
  parameter_selection/3(outport-mot4_ctrl_cstr_trq_max_pos_simu-3) -> mot4_ctrl_cmd_map_Pelec_funTW_volt_in/3(mot_ctrl_cstr_trq_max_pos_simu)
  parameter_selection/2(outport-mot4_ctrl_trs_trq_simu-2) -> mot4_ctrl_cmd_map_Pelec_funTW_volt_in/2(mot_ctrl_trs_trq_simu)
  parameter_selection/1(outport-mot4_plant_spd_out_simu-1) -> mot4_ctrl_cmd_map_Pelec_funTW_volt_in/1(mot_plant_spd_out_simu)
  mot4_ctrl_cmd_map_Pelec_funTW_volt_in/1(mot_ctrl_cmd_simu) -> parameter_out/1(inport-mot4_ctrl_cmd_simu)
  parameter_out/1(outport-system_info_bus) -> outport-system_info_bus/1
  inport-main_info_bus-1/1 -> parameter_selection/1(inport-main_info_bus-1)

== system AeroPropRefFranc/Propulsion and Aerodynamic Forces and Moments/S-Function/Battery Model/powerplant/mot4/ctrl/cstr ==
  inport-main_info_bus-1 : Inport
  aInport--2 : Inport  Port=2
  aInport--3 : Inport  Port=3
  Terminator_1 : Terminator
  Terminator_2 : Terminator
  mot4_ctrl_cstr_map_Pelec_funTW_volt_in : Subsystem
  parameter_out : Subsystem
  parameter_selection : Subsystem
  outport-system_info_bus : Outport
  outport-cstr_bus : Outport  Port=2
  wires:
  aInport--3/1 -> Terminator_2/1
  aInport--2/1 -> Terminator_1/1
  parameter_selection/2(outport-mot4_plant_temp_coeff_simu-2) -> mot4_ctrl_cstr_map_Pelec_funTW_volt_in/2(mot_plant_temp_coeff_simu)
  parameter_selection/1(outport-mot4_plant_spd_out_simu-1) -> mot4_ctrl_cstr_map_Pelec_funTW_volt_in/1(mot_plant_spd_out_simu)
  mot4_ctrl_cstr_map_Pelec_funTW_volt_in/7(mot_ctrl_cstr_temp_coeff_simu) -> parameter_out/7(inport-mot4_ctrl_cstr_temp_coeff_simu)
  mot4_ctrl_cstr_map_Pelec_funTW_volt_in/6(mot_ctrl_cstr_trq_cont_neg_simu) -> parameter_out/6(inport-mot4_ctrl_cstr_trq_cont_neg_simu)
  mot4_ctrl_cstr_map_Pelec_funTW_volt_in/5(mot_ctrl_cstr_trq_cont_pos_simu) -> parameter_out/5(inport-mot4_ctrl_cstr_trq_cont_pos_simu)
  mot4_ctrl_cstr_map_Pelec_funTW_volt_in/4(mot_ctrl_cstr_trq_max_neg_simu) -> parameter_out/4(inport-mot4_ctrl_cstr_trq_max_neg_simu)
  mot4_ctrl_cstr_map_Pelec_funTW_volt_in/3(mot_ctrl_cstr_trq_pk_neg_simu) -> parameter_out/3(inport-mot4_ctrl_cstr_trq_pk_neg_simu)
  mot4_ctrl_cstr_map_Pelec_funTW_volt_in/2(mot_ctrl_cstr_trq_max_pos_simu) -> parameter_out/2(inport-mot4_ctrl_cstr_trq_max_pos_simu)
  mot4_ctrl_cstr_map_Pelec_funTW_volt_in/1(mot_ctrl_cstr_trq_pk_pos_simu) -> parameter_out/1(inport-mot4_ctrl_cstr_trq_pk_pos_simu)
  parameter_out/2(outport-cstr_bus) -> outport-cstr_bus/1
  parameter_out/1(outport-system_info_bus) -> outport-system_info_bus/1
  inport-main_info_bus-1/1 -> parameter_selection/1(inport-main_info_bus-1)

== system AeroPropRefFranc/Propulsion and Aerodynamic Forces and Moments/S-Function/Battery Model/powerplant/mot4/ctrl/dmd ==
  inport-main_info_bus-1 : Inport
  aInport--2 : Inport  Port=2
  Terminator_1 : Terminator
  mot4_ctrl_dmd_uas : Subsystem
  parameter_out : Subsystem
  parameter_selection : Subsystem
  outport-system_info_bus : Outport
  outport-dmd_bus : Outport  Port=2
  wires:
  aInport--2/1 -> Terminator_1/1
  parameter_selection/5(outport-tc4_plant_spd_in_simu-5) -> mot4_ctrl_dmd_uas/5(tc_plant_spd_in_simu)
  parameter_selection/4(outport-propel4_plant_speed_simu-4) -> mot4_ctrl_dmd_uas/4(propel_plant_speed_simu)
  parameter_selection/3(outport-ess_ctrl_pwr_max_pro_simu-3) -> mot4_ctrl_dmd_uas/3(ess_ctrl_pwr_max_pro_simu)
  parameter_selection/2(outport-env_plant_density_simu-2) -> mot4_ctrl_dmd_uas/2(env_plant_density_simu)
  parameter_selection/1(outport-apc_ctrl_dt4_simu-1) -> mot4_ctrl_dmd_uas/1(apc_ctrl_dt_simu)
  mot4_ctrl_dmd_uas/2(mot_ctrl_ratedpwr_simu) -> parameter_out/2(inport-mot4_ctrl_ratedpwr_simu)
  mot4_ctrl_dmd_uas/1(mot_ctrl_trs_trq_simu) -> parameter_out/1(inport-mot4_ctrl_trs_trq_simu)
  parameter_out/2(outport-dmd_bus) -> outport-dmd_bus/1
  parameter_out/1(outport-system_info_bus) -> outport-system_info_bus/1
  inport-main_info_bus-1/1 -> parameter_selection/1(inport-main_info_bus-1)

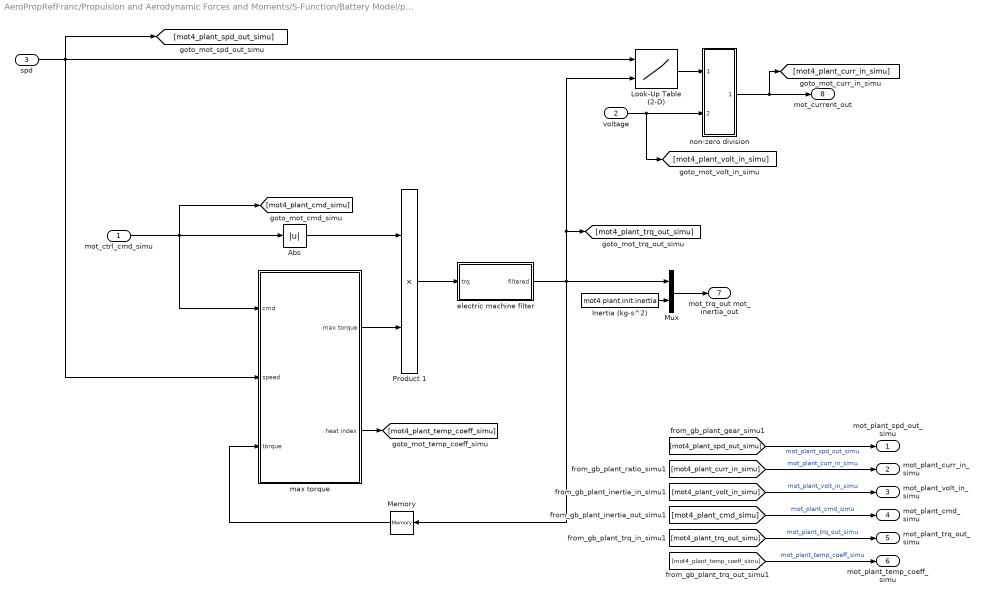
== system AeroPropRefFranc/Propulsion and Aerodynamic Forces and Moments/S-Function/Battery Model/powerplant/mot4/plant/mot4_plant_map_Pelec_funTW_volt_in ==
  mot_ctrl_cmd_simu : Inport
  voltage : Inport  Port=2
  spd : Inport  Port=3
  Abs : Abs
  Inertia (kg-s^2) : Constant  Value=mot4.plant.init.inertia
  Look-Up Table (2-D) : Lookup2D  RowIndex=mot4.plant.calc.pwr_elec.idx1_spd  ColumnIndex=mot4.plant.calc.pwr_elec.idx2_trq  Table=mot4.plant.calc.pwr_elec.map
  Memory : Memory
  Mux : Mux  Inputs=2
  Product 1 : Product  InputSameDT=on  SaturateOnIntegerOverflow=on  OutDataTypeStr=Inherit: Same as first input
  electric machine filter : Subsystem
  "max torque " : Subsystem
  non-zero division : Subsystem
      mask Display: disp('divider \n I1/I2')
  mot_plant_spd_out_simu : Outport
  mot_plant_curr_in_simu : Outport  Port=2
  mot_plant_volt_in_simu : Outport  Port=3
  mot_plant_cmd_simu : Outport  Port=4
  mot_plant_trq_out_simu : Outport  Port=5
  mot_plant_temp_coeff_simu : Outport  Port=6
  mot_trq_out mot_inertia_out : Outport  Port=7
  mot_current_out : Outport  Port=8
  wires:
  voltage/1 -> [mot4_plant_volt_in_simu], non-zero division/2(In2)
  non-zero division/1(Out1) -> [mot4_plant_curr_in_simu], mot_current_out/1
  "max torque "/2(heat index) -> [mot4_plant_temp_coeff_simu]
  spd/1 -> Look-Up Table (2-D)/1, "max torque "/2(speed), [mot4_plant_spd_out_simu]
  Mux/1 -> mot_trq_out mot_inertia_out/1
  Inertia (kg-s^2)/1 -> Mux/2
  mot_ctrl_cmd_simu/1 -> Abs/1, [mot4_plant_cmd_simu], "max torque "/1(cmd)
  Memory/1 -> "max torque "/3(torque)
  Abs/1 -> Product 1/1
  Product 1/1 -> electric machine filter/1(trq)
  "max torque "/1(max torque) -> Product 1/2
  electric machine filter/1(filtered) -> Look-Up Table (2-D)/2, [mot4_plant_trq_out_simu], Memory/1, Mux/1
  [mot4_plant_spd_out_simu] -> mot_plant_spd_out_simu/1  "mot_plant_spd_out_simu"
  [mot4_plant_curr_in_simu] -> mot_plant_curr_in_simu/1  "mot_plant_curr_in_simu"
  [mot4_plant_volt_in_simu] -> mot_plant_volt_in_simu/1  "mot_plant_volt_in_simu"
  [mot4_plant_cmd_simu] -> mot_plant_cmd_simu/1  "mot_plant_cmd_simu"
  [mot4_plant_trq_out_simu] -> mot_plant_trq_out_simu/1  "mot_plant_trq_out_simu"
  [mot4_plant_temp_coeff_simu] -> mot_plant_temp_coeff_simu/1  "mot_plant_temp_coeff_simu"
  Look-Up Table (2-D)/1 -> non-zero division/1(In1)

== system AeroPropRefFranc/Propulsion and Aerodynamic Forces and Moments/S-Function/Battery Model/powerplant/mot4/plant/parameter_out ==
  inport-mot4_plant_spd_out_simu : Inport
  inport-mot4_plant_curr_in_simu : Inport  Port=2
  inport-mot4_plant_volt_in_simu : Inport  Port=3
  inport-mot4_plant_cmd_simu : Inport  Port=4
  inport-mot4_plant_trq_out_simu : Inport  Port=5
  inport-mot4_plant_temp_coeff_simu : Inport  Port=6
  Ground_1 : Ground
  Toworkspace-mot4_plant_cmd_simu : ToWorkspace  VariableName=mot4_plant_cmd_simu  SampleTime=pxf_diagram_options.workspace_sample_time
      settings: Decimation=pxf_diagram_options.decimation
  Toworkspace-mot4_plant_curr_in_simu : ToWorkspace  VariableName=mot4_plant_curr_in_simu  SampleTime=pxf_diagram_options.workspace_sample_time
      settings: Decimation=pxf_diagram_options.decimation
  Toworkspace-mot4_plant_spd_out_simu : ToWorkspace  VariableName=mot4_plant_spd_out_simu  SampleTime=pxf_diagram_options.workspace_sample_time
      settings: Decimation=pxf_diagram_options.decimation
  Toworkspace-mot4_plant_temp_coeff_simu : ToWorkspace  VariableName=mot4_plant_temp_coeff_simu  SampleTime=pxf_diagram_options.workspace_sample_time
      settings: Decimation=pxf_diagram_options.decimation
  Toworkspace-mot4_plant_trq_out_simu : ToWorkspace  VariableName=mot4_plant_trq_out_simu  SampleTime=pxf_diagram_options.workspace_sample_time
      settings: Decimation=pxf_diagram_options.decimation
  Toworkspace-mot4_plant_volt_in_simu : ToWorkspace  VariableName=mot4_plant_volt_in_simu  SampleTime=pxf_diagram_options.workspace_sample_time
      settings: Decimation=pxf_diagram_options.decimation
  create_system_info_bus : BusCreator  Inputs=2
  outport-system_info_bus : Outport
  outport-plant_bus : Outport  Port=2
  wires:
  Ground_1/1 -> outport-plant_bus/1
  inport-mot4_plant_temp_coeff_simu/1 -> Toworkspace-mot4_plant_temp_coeff_simu/1, create_system_info_bus/2  "mot4_plant_temp_coeff_simu"
  inport-mot4_plant_trq_out_simu/1 -> Toworkspace-mot4_plant_trq_out_simu/1
  inport-mot4_plant_cmd_simu/1 -> Toworkspace-mot4_plant_cmd_simu/1
  inport-mot4_plant_volt_in_simu/1 -> Toworkspace-mot4_plant_volt_in_simu/1
  inport-mot4_plant_curr_in_simu/1 -> Toworkspace-mot4_plant_curr_in_simu/1
  inport-mot4_plant_spd_out_simu/1 -> Toworkspace-mot4_plant_spd_out_simu/1, create_system_info_bus/1  "mot4_plant_spd_out_simu"
  create_system_info_bus/1 -> outport-system_info_bus/1

== system AeroPropRefFranc/Propulsion and Aerodynamic Forces and Moments/S-Function/Battery Model/powerplant/mot4/plant/parameter_selection ==
  Inport_1 : Inport
  inport-ctrl_bus-2 : Inport  Port=2
  Terminator_1 : Terminator
  select_ctrl_bus : BusSelector  OutputSignals=mot4_ctrl_cmd_simu
  outport-mot4_ctrl_cmd_simu-1 : Outport
  wires:
  Inport_1/1 -> Terminator_1/1
  select_ctrl_bus/1 -> outport-mot4_ctrl_cmd_simu-1/1  "<mot4_ctrl_cmd_simu>"
  inport-ctrl_bus-2/1 -> select_ctrl_bus/1

== system AeroPropRefFranc/Propulsion and Aerodynamic Forces and Moments/S-Function/Battery Model/powerplant/propel/plant/parameter_out ==
  inport-propel_plant_speed_simu : Inport
  inport-propel_plant_pwr_in_simu : Inport  Port=2
  inport-propel_plant_pwr_out_simu : Inport  Port=3
  inport-propel_plant_thrust_simu : Inport  Port=4
  Toworkspace-propel_plant_pwr_in_simu : ToWorkspace  VariableName=propel_plant_pwr_in_simu  SampleTime=pxf_diagram_options.workspace_sample_time
      settings: Decimation=pxf_diagram_options.decimation
  Toworkspace-propel_plant_pwr_out_simu : ToWorkspace  VariableName=propel_plant_pwr_out_simu  SampleTime=pxf_diagram_options.workspace_sample_time
      settings: Decimation=pxf_diagram_options.decimation
  Toworkspace-propel_plant_speed_simu : ToWorkspace  VariableName=propel_plant_speed_simu  SampleTime=pxf_diagram_options.workspace_sample_time
      settings: Decimation=pxf_diagram_options.decimation
  Toworkspace-propel_plant_thrust_simu : ToWorkspace  VariableName=propel_plant_thrust_simu  SampleTime=pxf_diagram_options.workspace_sample_time
      settings: Decimation=pxf_diagram_options.decimation
  create_system_info_bus : BusCreator  Inputs=1
  outport-system_info_bus : Outport
  wires:
  inport-propel_plant_thrust_simu/1 -> Toworkspace-propel_plant_thrust_simu/1
  inport-propel_plant_pwr_out_simu/1 -> Toworkspace-propel_plant_pwr_out_simu/1
  inport-propel_plant_pwr_in_simu/1 -> Toworkspace-propel_plant_pwr_in_simu/1
  inport-propel_plant_speed_simu/1 -> Toworkspace-propel_plant_speed_simu/1, create_system_info_bus/1  "propel_plant_speed_simu"
  create_system_info_bus/1 -> outport-system_info_bus/1

== system AeroPropRefFranc/Propulsion and Aerodynamic Forces and Moments/S-Function/Battery Model/powerplant/propel/plant/parameter_selection ==
  inport-main_info_bus-1 : Inport
  select_main_info_bus : BusSelector  OutputSignals=env_info_bus.env_plant_density_simu,apa_info_bus.powerplant_info_bus.tc.tc_plant_inertia_out_simu,apa_info_bus.apa_plant_info_bus.apa_plant_info_bus.forceeq_bus.eqnmotion_plant_linvel_simu
  outport-env_plant_density_simu-1 : Outport
  outport-tc_plant_inertia_out_simu-2 : Outport  Port=2
  outport-eqnmotion_plant_linvel_simu-3 : Outport  Port=3
  wires:
  select_main_info_bus/3 -> outport-eqnmotion_plant_linvel_simu-3/1  "<eqnmotion_plant_linvel_simu>"
  select_main_info_bus/2 -> outport-tc_plant_inertia_out_simu-2/1  "<tc_plant_inertia_out_simu>"
  select_main_info_bus/1 -> outport-env_plant_density_simu-1/1  "<env_plant_density_simu>"
  inport-main_info_bus-1/1 -> select_main_info_bus/1

== system AeroPropRefFranc/Propulsion and Aerodynamic Forces and Moments/S-Function/Battery Model/powerplant/propel/plant/propel_plant_uas ==
  note: rev/s
  note: rad/s
  env_plant_density_simu : Inport
  tc_plant_inertia_out_simu : Inport  Port=2
  eqnmotion_plant_linvel_simu : Inport  Port=3
  tc_plant_trq_out_simu : Inport  Port=4
  flow-in : Inport  Port=5
  Gain : Gain  Gain=propel.plant.init.thrustdir
  Gain1 : Gain  Gain=2*pi
  Gain2 : Gain
  Gain3 : Gain
  Mux : Mux  Inputs=2
  Propeller Power : Subsystem
  Propeller_CP : Subsystem
  Propeller_Torque : Subsystem
  Terminator : Terminator
  Thrust_Generated : Subsystem
  Total_Moment : Subsystem
  propel_plant_speed_simu : Outport  VectorParamsAs1DForOutWhenUnconnected=off
  propel_plant_pwr_in_simu : Outport  Port=2  VectorParamsAs1DForOutWhenUnconnected=off
  propel_plant_pwr_out_simu : Outport  Port=3  VectorParamsAs1DForOutWhenUnconnected=off
  propel_plant_thrust_simu : Outport  Port=4  VectorParamsAs1DForOutWhenUnconnected=off
  propel_plant_effort : Outport  Port=5  VectorParamsAs1DForOutWhenUnconnected=off
  propel_plant_speed_out_simu : Outport  Port=6  VectorParamsAs1DForOutWhenUnconnected=off
  wires:
  Thrust_Generated/1(propel_plant_thrust_simu) -> propel_plant_thrust_simu/1, Gain/1, Total_Moment/1(propel_plant_thrust_simu), Propeller Power/3(propel_plant_thrust_simu)  "propel_plant_thrust_simu"
  Propeller_Torque/1(propel_plant_rps_simu) -> Thrust_Generated/2(propel_plant_speed_simu), Propeller_CP/1(propel_plant_rps_simu), Gain1/1, Propeller Power/4(propel_plant_rps_simu)
  Propeller_CP/1(propel_plant_CP_simu) -> Propeller_Torque/2(propel_plant_CP_simu), Propeller Power/2(propel_plant_CP_simu)
  Thrust_Generated/2(propel_plant_CT_simu) -> Propeller Power/1(propel_plant_CT_simu)
  env_plant_density_simu/1 -> Propeller_Torque/1(env_plant_density_simu), Thrust_Generated/1(env_plant_density_simu)
  tc_plant_trq_out_simu/1 -> Propeller_Torque/3(tc_plant_trq_out_simu)
  tc_plant_inertia_out_simu/1 -> Propeller_Torque/4(tc_plant_inertia_out_simu)
  Total_Moment/1(accmoment_plant_totmoment_simu) -> Mux/2  "effort_plant_angleffort_simu"
  Propeller_Torque/2(propel_plant_restq_simu) -> Total_Moment/2(propel_plant_restq_simu)
  Gain/1 -> Mux/1  "effort_plant_longeffort_simu"
  Mux/1 -> propel_plant_effort/1  "propel_plant_effort"
  eqnmotion_plant_linvel_simu/1 -> Propeller Power/5(eqnmotion_plant_linvel_simu)
  Gain1/1 -> Gain3/1, Gain2/1
  Propeller Power/2(propel_plant_pwr_out_simu) -> propel_plant_pwr_out_simu/1  "propel_plant_pwr_out_simu"
  Propeller Power/1(propel_plant_pwr_in_simu) -> propel_plant_pwr_in_simu/1  "propel_plant_pwr_in_simu"
  Gain2/1 -> propel_plant_speed_out_simu/1  "propel_plant_speed_out_simu"
  Gain3/1 -> propel_plant_speed_simu/1  "propel_plant_speed_simu"
  flow-in/1 -> Terminator/1
